simulink library "csu_tracker_mcu_signal_interface_lib"  (R2014b)
settings: Solver=ode45  StartTime=0.0  StopTime=10.0  RelTol=1e-3
libraries: util_info_lib x1
settings Model: Creator=escrane  LastModifiedBy=mstewart

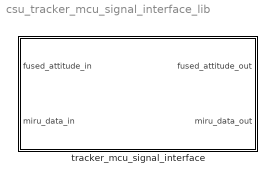
== system csu_tracker_mcu_signal_interface_lib ==
  tracker_mcu_signal_interface : Subsystem

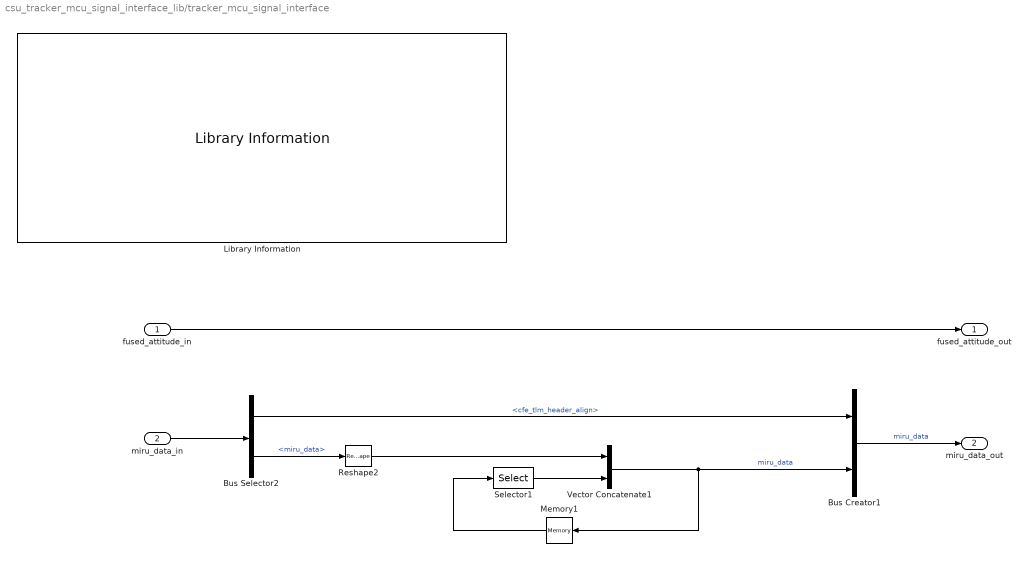
== system csu_tracker_mcu_signal_interface_lib/tracker_mcu_signal_interface ==
  fused_attitude_in : Inport
  miru_data_in : Inport  Port=2
  Bus Selector2 : BusSelector  OutputSignals=cfe_tlm_header_align,miru_data
  Bus Creator1 : BusCreator  Inputs=2
  Library Information : util_info_lib/Library Information  owner='NONE'
  Memory1 : Memory  X0=zeros(10,11)  InheritSampleTime=on
  Reshape2 : Reshape  OutputDimensionality=Row vector (2-D)
  Selector1 : Selector  NumberOfDimensions=2  InputPortWidth=10  IndexOptions=Index vector (dialog),Select all  Indices=[1:9],1  OutputSizes=1,1
  Vector Concatenate1 : Concatenate  Mode=Multidimensional array
  fused_attitude_out : Outport
  miru_data_out : Outport  Port=2
  wires:
  Bus Selector2/1 -> Bus Creator1/1  "<cfe_tlm_header_align>"
  Bus Creator1/1 -> miru_data_out/1  "miru_data"
  fused_attitude_in/1 -> fused_attitude_out/1
  Bus Selector2/2 -> Reshape2/1  "<miru_data>"
  miru_data_in/1 -> Bus Selector2/1
  Memory1/1 -> Selector1/1
  Selector1/1 -> Vector Concatenate1/2
  Vector Concatenate1/1 -> Bus Creator1/2, Memory1/1  "miru_data"
  Reshape2/1 -> Vector Concatenate1/1
